simulink model "dropletdet"  (R2012b)
settings: Solver=ode45  SolverMode=SingleTasking  StartTime=0.0  StopTime=43002  RelTol=1e-3
libraries: xbsIndex_r4 x253, simulink x1
(part 1 of 2)
settings Model: Creator=skhay  LastModifiedBy=casrm

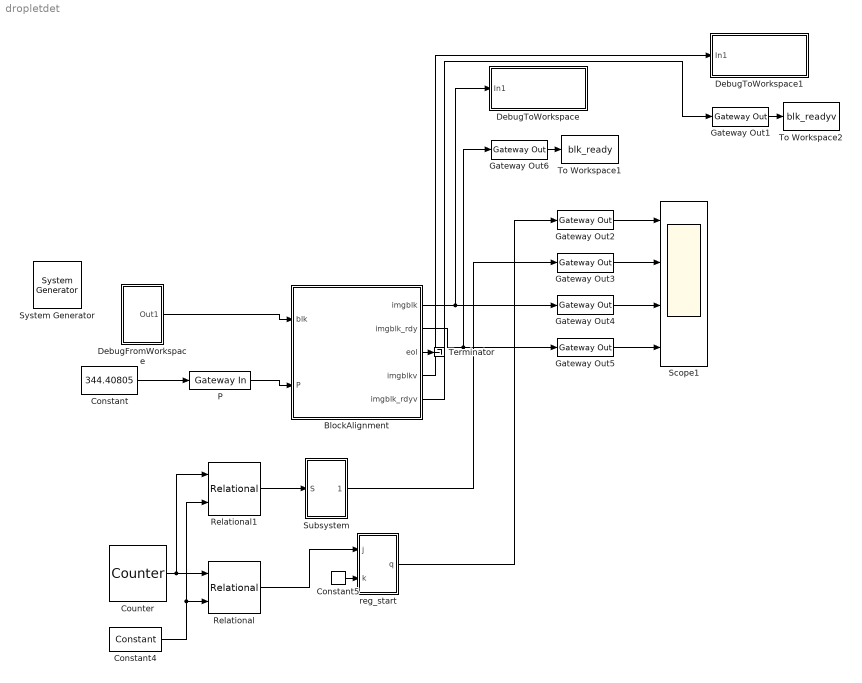
== system dropletdet ==
  " System Generator" : xbsIndex_r4/ System Generator  Tag=genX  xilinxfamily=virtex6  part=xc6vsx475t  speed=-1  package=ff1759  synthesis_tool=XST  clock_wrapper=Clock Enables  directory=./celldet_ppp_sysgen  proj_type=Project Navigator  Synth_file=XST Defaults  Impl_file=ISE Defaults  testbench=off  simulink_period=1  sysclk_period=5  dcm_input_clock_period=100  incr_netlist=off  trim_vbits=Everywhere in SubSystem  dbl_ovrd=According to Block Masks  core_generation=According to Block Masks  run_coregen=off  deprecated_control=off  eval_field=0  block_type=sysgen
      settings: block_version=11.4
  BlockAlignment : Subsystem
  Constant : Constant  Value=344.40805
  Constant4 : xbsIndex_r4/Constant  const=100  gui_display_data_type=Fixed-point  arith_type=Unsigned  n_bits=8  bin_pt=0  preci_type=Single  exp_width=8  frac_width=24  explicit_period=off  period=1  equ=P=C  opselect=C  inp2=PCIN>>17  opr=+  inp1=P  carry=CIN  dbl_ovrd=off  block_type=constant
  Constant5 : xbsIndex_r4/Constant  const=0  gui_display_data_type=Boolean  arith_type=Boolean  n_bits=16  bin_pt=14  preci_type=Single  exp_width=8  frac_width=24  explicit_period=off  period=1  equ=P=C  opselect=C  inp2=PCIN>>17  opr=+  inp1=P  carry=CIN  dbl_ovrd=off  block_type=constant
  Counter : xbsIndex_r4/Counter  cnt_type=Free Running  cnt_to=255  operation=Up  start_count=0  cnt_by_val=1  arith_type=Unsigned  n_bits=8  bin_pt=0  load_pin=off  rst=off  en=off  explicit_period=on  period=1  dbl_ovrd=off  use_behavioral_HDL=off  implementation=Fabric  block_type=counter
  DebugFromWorkspace : Subsystem
  DebugToWorkspace : Subsystem
  DebugToWorkspace1 : Subsystem
  Gateway Out1 : xbsIndex_r4/Gateway Out  inherit_from_input=on  hdl_port=off  timing_constraint=None  locs_specified=off  LOCs={}  UseAsDAC=off  DACChannel='1'  block_type=gatewayout
  Gateway Out{2..5} (4 alike) : xbsIndex_r4/Gateway Out  inherit_from_input=off  hdl_port=off  timing_constraint=None  locs_specified=off  LOCs={}  UseAsDAC=off  DACChannel='1'  block_type=gatewayout
  Gateway Out6 : xbsIndex_r4/Gateway Out  inherit_from_input=on  hdl_port=off  timing_constraint=None  locs_specified=off  LOCs={}  UseAsDAC=off  DACChannel='1'  block_type=gatewayout
  P : xbsIndex_r4/Gateway In  gui_display_data_type=Fixed-point  arith_type=Unsigned  n_bits=32  bin_pt=20  preci_type=Single  exp_width=8  frac_width=24  quantization="Round  (unbiased: +/- Inf)"  overflow=Saturate  period=1  dbl_ovrd=off  timing_constraint=None  locs_specified=off  LOCs={}  UseAsADC=off  ADCChannel='1'  inherit_from_input=off  hdl_port=on  block_type=gatewayin
  Relational : xbsIndex_r4/Relational  mode=a>b  en=off  latency=0  dbl_ovrd=off  block_type=relational
  Relational1 : xbsIndex_r4/Relational  mode=a=b  en=off  latency=0  dbl_ovrd=off  block_type=relational
  Scope1 : Scope  NumInputPorts=4
      settings: YMin=-5~-5~-5~-5  YMax=5~5~5~5  SaveName=ScopeData7
  Subsystem : Subsystem
  Terminator : Terminator
  To Workspace1 : ToWorkspace  VariableName=blk_ready  SampleTime=-1
  To Workspace2 : ToWorkspace  VariableName=blk_readyv  SampleTime=-1
  reg_start : Subsystem
  wires:
  P/1 -> BlockAlignment/2(P)
  Constant/1 -> P/1
  DebugFromWorkspace/1(Out1) -> BlockAlignment/1(blk)
  BlockAlignment/1(imgblk) -> DebugToWorkspace/1(In1), Gateway Out4/1
  BlockAlignment/2(imgblk_rdy) -> Gateway Out6/1, Gateway Out5/1
  BlockAlignment/3(eol) -> Terminator/1
  Counter/1 -> Relational1/1, Relational/1
  Constant4/1 -> Relational1/2, Relational/2
  reg_start/1(q) -> Gateway Out2/1
  Gateway Out5/1 -> Scope1/4
  Gateway Out4/1 -> Scope1/3
  Gateway Out3/1 -> Scope1/2
  Gateway Out2/1 -> Scope1/1
  Relational/1 -> reg_start/1(j)
  Constant5/1 -> reg_start/2(k)
  Subsystem/1(start) -> Gateway Out3/1
  Relational1/1 -> Subsystem/1(S)
  Gateway Out6/1 -> To Workspace1/1
  BlockAlignment/4(imgblkv) -> DebugToWorkspace1/1(In1)
  BlockAlignment/5(imgblk_rdyv) -> Gateway Out1/1
  Gateway Out1/1 -> To Workspace2/1

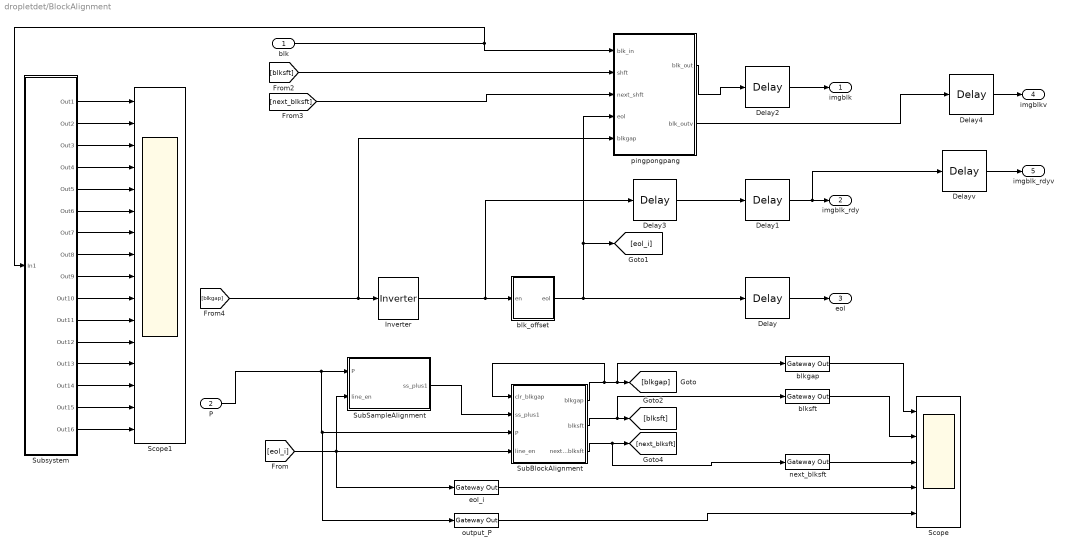
== system dropletdet/BlockAlignment ==
  blk : Inport
  P : Inport  Port=2
  Delay{,1..4} (5 alike) : xbsIndex_r4/Delay  rst=off  infoeditControl=Selection of Reset will increase slice count due to use of real FFs and instead of SRLs  en=off  latency=1  dbl_ovrd=off  reg_retiming=off  block_type=delay
  Delayv : xbsIndex_r4/Delay  rst=off  infoeditControl=Selection of Reset will increase slice count due to use of real FFs and instead of SRLs  en=off  latency=10  dbl_ovrd=off  reg_retiming=off  block_type=delay
  Inverter : xbsIndex_r4/Inverter  en=off  latency=0  dbl_ovrd=off  block_type=inv
  Scope : Scope  NumInputPorts=5
      settings: ShowLegends=on  TimeRange=2102  YMin=-5~-5~-5~-5~-5  YMax=5~5~20~5~5  SaveName=ScopeData4
  Scope1 : Scope  NumInputPorts=16
      settings: TimeRange=2102  YMin=-5~-5~-5~-5~-5~-5~-5~-5~-5~-5~-5~-5~-5~-5~-5~-5  YMax=5~5~20~5~5~5~5~5~5~5~5~5~5~5~5~5  SaveName=ScopeData6
  SubBlockAlignment : Subsystem
  SubSampleAlignment : Subsystem
  Subsystem : Subsystem
  blk_offset : Subsystem
  blkgap : xbsIndex_r4/Gateway Out  inherit_from_input=off  hdl_port=off  timing_constraint=None  locs_specified=off  LOCs={}  UseAsDAC=off  DACChannel='1'  block_type=gatewayout
  blksft : xbsIndex_r4/Gateway Out  inherit_from_input=off  hdl_port=off  timing_constraint=None  locs_specified=off  LOCs={}  UseAsDAC=off  DACChannel='1'  block_type=gatewayout
  eol_i : xbsIndex_r4/Gateway Out  inherit_from_input=off  hdl_port=off  timing_constraint=None  locs_specified=off  LOCs={}  UseAsDAC=off  DACChannel='1'  block_type=gatewayout
  next_blksft : xbsIndex_r4/Gateway Out  inherit_from_input=off  hdl_port=off  timing_constraint=None  locs_specified=off  LOCs={}  UseAsDAC=off  DACChannel='1'  block_type=gatewayout
  output_P : xbsIndex_r4/Gateway Out  inherit_from_input=off  hdl_port=off  timing_constraint=None  locs_specified=off  LOCs={}  UseAsDAC=off  DACChannel='1'  block_type=gatewayout
  pingpongpang : Subsystem
  imgblk : Outport
  imgblk_rdy : Outport  Port=2
  eol : Outport  Port=3
  imgblkv : Outport  Port=4
  imgblk_rdyv : Outport  Port=5
  wires:
  [blkgap] -> pingpongpang/5(blkgap), Inverter/1
  Delay/1 -> eol/1
  [blksft] -> pingpongpang/2(shft)
  [next_blksft] -> pingpongpang/3(next_shft)
  P/1 -> output_P/1, SubBlockAlignment/3(P), SubSampleAlignment/1(P)
  SubSampleAlignment/1(ss_plus1) -> SubBlockAlignment/2(ss_plus1)
  SubBlockAlignment/1(blkgap) -> SubBlockAlignment/1(clr_blkgap), blkgap/1, [blkgap]
  SubBlockAlignment/2(blksft) -> blksft/1, [blksft]
  SubBlockAlignment/3(next_blksft) -> next_blksft/1, [next_blksft]
  [eol_i] -> eol_i/1, SubSampleAlignment/2(line_en), SubBlockAlignment/4(line_en)
  blk/1 -> Subsystem/1(In1), pingpongpang/1(blk_in)
  Delay2/1 -> imgblk/1
  blk_offset/1(eol) -> pingpongpang/4(eol), [eol_i], Delay/1
  Delay1/1 -> Delayv/1, imgblk_rdy/1
  blkgap/1 -> Scope/1
  blksft/1 -> Scope/2
  next_blksft/1 -> Scope/3
  eol_i/1 -> Scope/4
  Inverter/1 -> Delay3/1, blk_offset/1(en)
  Delay3/1 -> Delay1/1
  Subsystem/1(Out1) -> Scope1/1
  Subsystem/2(Out2) -> Scope1/2
  Subsystem/3(Out3) -> Scope1/3
  Subsystem/4(Out4) -> Scope1/4
  Subsystem/5(Out5) -> Scope1/5
  Subsystem/6(Out6) -> Scope1/6
  Subsystem/7(Out7) -> Scope1/7
  Subsystem/8(Out8) -> Scope1/8
  Subsystem/9(Out9) -> Scope1/9
  Subsystem/10(Out10) -> Scope1/10
  Subsystem/11(Out11) -> Scope1/11
  Subsystem/12(Out12) -> Scope1/12
  Subsystem/13(Out13) -> Scope1/13
  Subsystem/14(Out14) -> Scope1/14
  Subsystem/15(Out15) -> Scope1/15
  Subsystem/16(Out16) -> Scope1/16
  output_P/1 -> Scope/5
  Delay4/1 -> imgblkv/1
  pingpongpang/1(blk_out) -> Delay2/1
  Delayv/1 -> imgblk_rdyv/1
  pingpongpang/2(blk_outv) -> Delay4/1

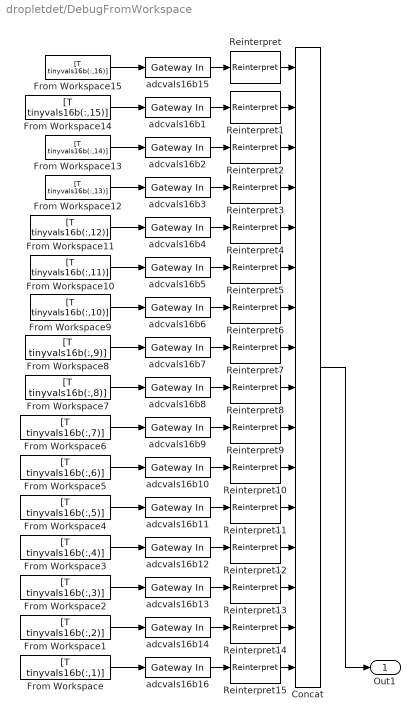
== system dropletdet/DebugFromWorkspace ==
  Concat : xbsIndex_r4/Concat  num_inputs=16  dbl_ovrd=off  block_type=concat
  From Workspace : FromWorkspace  VariableName=[T tinyvals16b(:,1)]  SampleTime=1
  From Workspace1 : FromWorkspace  VariableName=[T tinyvals16b(:,2)]  SampleTime=1
  From Workspace10 : FromWorkspace  VariableName=[T tinyvals16b(:,11)]  SampleTime=1
  From Workspace11 : FromWorkspace  VariableName=[T tinyvals16b(:,12)]  SampleTime=1
  From Workspace12 : FromWorkspace  VariableName=[T tinyvals16b(:,13)]  SampleTime=1
  From Workspace13 : FromWorkspace  VariableName=[T tinyvals16b(:,14)]  SampleTime=1
  From Workspace14 : FromWorkspace  VariableName=[T tinyvals16b(:,15)]  SampleTime=1
  From Workspace15 : FromWorkspace  VariableName=[T tinyvals16b(:,16)]  SampleTime=1
  From Workspace2 : FromWorkspace  VariableName=[T tinyvals16b(:,3)]  SampleTime=1
  From Workspace3 : FromWorkspace  VariableName=[T tinyvals16b(:,4)]  SampleTime=1
  From Workspace4 : FromWorkspace  VariableName=[T tinyvals16b(:,5)]  SampleTime=1
  From Workspace5 : FromWorkspace  VariableName=[T tinyvals16b(:,6)]  SampleTime=1
  From Workspace6 : FromWorkspace  VariableName=[T tinyvals16b(:,7)]  SampleTime=1
  From Workspace7 : FromWorkspace  VariableName=[T tinyvals16b(:,8)]  SampleTime=1
  From Workspace8 : FromWorkspace  VariableName=[T tinyvals16b(:,9)]  SampleTime=1
  From Workspace9 : FromWorkspace  VariableName=[T tinyvals16b(:,10)]  SampleTime=1
  Reinterpret{,1..15} (16 alike) : xbsIndex_r4/Reinterpret  force_arith_type=on  arith_type=Unsigned  force_bin_pt=on  bin_pt=0  block_type=reinterpret
  adcvals16b{1..16} (16 alike) : xbsIndex_r4/Gateway In  gui_display_data_type=Fixed-point  arith_type="Signed  (2's comp)"  n_bits=8  bin_pt=0  preci_type=Single  exp_width=8  frac_width=24  quantization="Round  (unbiased: +/- Inf)"  overflow=Saturate  period=1  dbl_ovrd=off  timing_constraint=None  locs_specified=off  LOCs={}  UseAsADC=off  ADCChannel='1'  inherit_from_input=off  hdl_port=on  block_type=gatewayin
  Out1 : Outport
  wires:
  Concat/1 -> Out1/1
  From Workspace15/1 -> adcvals16b15/1
  From Workspace14/1 -> adcvals16b1/1
  From Workspace13/1 -> adcvals16b2/1
  From Workspace12/1 -> adcvals16b3/1
  From Workspace11/1 -> adcvals16b4/1
  From Workspace10/1 -> adcvals16b5/1
  From Workspace9/1 -> adcvals16b6/1
  From Workspace8/1 -> adcvals16b7/1
  From Workspace7/1 -> adcvals16b8/1
  From Workspace6/1 -> adcvals16b9/1
  From Workspace5/1 -> adcvals16b10/1
  From Workspace4/1 -> adcvals16b11/1
  From Workspace3/1 -> adcvals16b12/1
  From Workspace2/1 -> adcvals16b13/1
  From Workspace1/1 -> adcvals16b14/1
  From Workspace/1 -> adcvals16b16/1
  adcvals16b15/1 -> Reinterpret/1
  Reinterpret/1 -> Concat/1
  adcvals16b1/1 -> Reinterpret1/1
  Reinterpret1/1 -> Concat/2
  adcvals16b2/1 -> Reinterpret2/1
  Reinterpret2/1 -> Concat/3
  adcvals16b3/1 -> Reinterpret3/1
  Reinterpret3/1 -> Concat/4
  adcvals16b4/1 -> Reinterpret4/1
  Reinterpret4/1 -> Concat/5
  adcvals16b5/1 -> Reinterpret5/1
  Reinterpret5/1 -> Concat/6
  adcvals16b6/1 -> Reinterpret6/1
  Reinterpret6/1 -> Concat/7
  adcvals16b7/1 -> Reinterpret7/1
  Reinterpret7/1 -> Concat/8
  adcvals16b8/1 -> Reinterpret8/1
  Reinterpret8/1 -> Concat/9
  adcvals16b9/1 -> Reinterpret9/1
  Reinterpret9/1 -> Concat/10
  adcvals16b10/1 -> Reinterpret10/1
  Reinterpret10/1 -> Concat/11
  adcvals16b11/1 -> Reinterpret11/1
  Reinterpret11/1 -> Concat/12
  adcvals16b12/1 -> Reinterpret12/1
  Reinterpret12/1 -> Concat/13
  adcvals16b13/1 -> Reinterpret13/1
  Reinterpret13/1 -> Concat/14
  adcvals16b14/1 -> Reinterpret14/1
  Reinterpret14/1 -> Concat/15
  adcvals16b16/1 -> Reinterpret15/1
  Reinterpret15/1 -> Concat/16

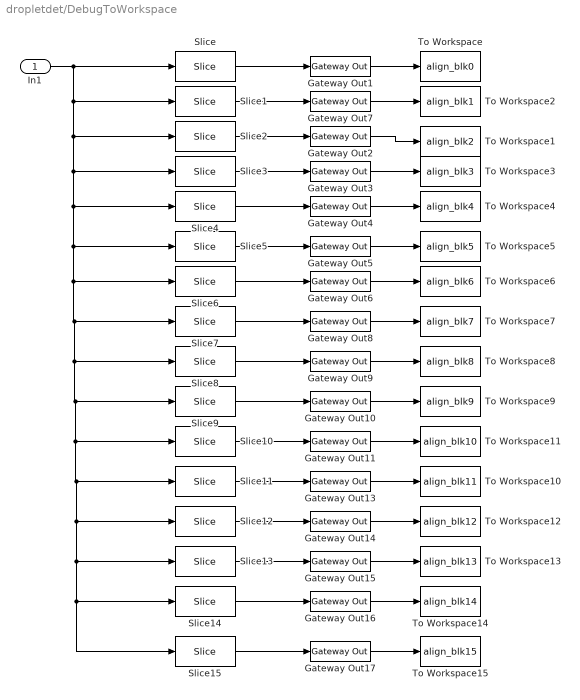
== system dropletdet/DebugToWorkspace ==
  In1 : Inport
  Gateway Out{1..11,13..17} (16 alike) : xbsIndex_r4/Gateway Out  inherit_from_input=on  hdl_port=off  timing_constraint=None  locs_specified=off  LOCs={}  UseAsDAC=off  DACChannel='1'  block_type=gatewayout
  Slice : xbsIndex_r4/Slice  nbits=8  boolean_output=off  mode=Lower Bit Location + Width  bit1=120  base1=MSB of Input  bit0=0  base0=LSB of Input  dbl_ovrd=off  block_type=slice
  Slice1 : xbsIndex_r4/Slice  nbits=8  boolean_output=off  mode=Lower Bit Location + Width  bit1=120  base1=MSB of Input  bit0=8  base0=LSB of Input  dbl_ovrd=off  block_type=slice
  Slice10 : xbsIndex_r4/Slice  nbits=8  boolean_output=off  mode=Lower Bit Location + Width  bit1=120  base1=MSB of Input  bit0=80  base0=LSB of Input  dbl_ovrd=off  block_type=slice
  Slice11 : xbsIndex_r4/Slice  nbits=8  boolean_output=off  mode=Lower Bit Location + Width  bit1=120  base1=MSB of Input  bit0=88  base0=LSB of Input  dbl_ovrd=off  block_type=slice
  Slice12 : xbsIndex_r4/Slice  nbits=8  boolean_output=off  mode=Lower Bit Location + Width  bit1=120  base1=MSB of Input  bit0=96  base0=LSB of Input  dbl_ovrd=off  block_type=slice
  Slice13 : xbsIndex_r4/Slice  nbits=8  boolean_output=off  mode=Lower Bit Location + Width  bit1=120  base1=MSB of Input  bit0=104  base0=LSB of Input  dbl_ovrd=off  block_type=slice
  Slice14 : xbsIndex_r4/Slice  nbits=8  boolean_output=off  mode=Lower Bit Location + Width  bit1=120  base1=MSB of Input  bit0=112  base0=LSB of Input  dbl_ovrd=off  block_type=slice
  Slice15 : xbsIndex_r4/Slice  nbits=8  boolean_output=off  mode=Lower Bit Location + Width  bit1=120  base1=MSB of Input  bit0=120  base0=LSB of Input  dbl_ovrd=off  block_type=slice
  Slice2 : xbsIndex_r4/Slice  nbits=8  boolean_output=off  mode=Lower Bit Location + Width  bit1=120  base1=MSB of Input  bit0=16  base0=LSB of Input  dbl_ovrd=off  block_type=slice
  Slice3 : xbsIndex_r4/Slice  nbits=8  boolean_output=off  mode=Lower Bit Location + Width  bit1=120  base1=MSB of Input  bit0=24  base0=LSB of Input  dbl_ovrd=off  block_type=slice
  Slice4 : xbsIndex_r4/Slice  nbits=8  boolean_output=off  mode=Lower Bit Location + Width  bit1=120  base1=MSB of Input  bit0=32  base0=LSB of Input  dbl_ovrd=off  block_type=slice
  Slice5 : xbsIndex_r4/Slice  nbits=8  boolean_output=off  mode=Lower Bit Location + Width  bit1=120  base1=MSB of Input  bit0=40  base0=LSB of Input  dbl_ovrd=off  block_type=slice
  Slice6 : xbsIndex_r4/Slice  nbits=8  boolean_output=off  mode=Lower Bit Location + Width  bit1=120  base1=MSB of Input  bit0=48  base0=LSB of Input  dbl_ovrd=off  block_type=slice
  Slice7 : xbsIndex_r4/Slice  nbits=8  boolean_output=off  mode=Lower Bit Location + Width  bit1=120  base1=MSB of Input  bit0=56  base0=LSB of Input  dbl_ovrd=off  block_type=slice
  Slice8 : xbsIndex_r4/Slice  nbits=8  boolean_output=off  mode=Lower Bit Location + Width  bit1=120  base1=MSB of Input  bit0=64  base0=LSB of Input  dbl_ovrd=off  block_type=slice
  Slice9 : xbsIndex_r4/Slice  nbits=8  boolean_output=off  mode=Lower Bit Location + Width  bit1=120  base1=MSB of Input  bit0=72  base0=LSB of Input  dbl_ovrd=off  block_type=slice
  To Workspace : ToWorkspace  VariableName=align_blk0  SampleTime=-1
  To Workspace1 : ToWorkspace  VariableName=align_blk2  SampleTime=-1
  To Workspace10 : ToWorkspace  VariableName=align_blk11  SampleTime=-1
  To Workspace11 : ToWorkspace  VariableName=align_blk10  SampleTime=-1
  To Workspace12 : ToWorkspace  VariableName=align_blk12  SampleTime=-1
  To Workspace13 : ToWorkspace  VariableName=align_blk13  SampleTime=-1
  To Workspace14 : ToWorkspace  VariableName=align_blk14  SampleTime=-1
  To Workspace15 : ToWorkspace  VariableName=align_blk15  SampleTime=-1
  To Workspace2 : ToWorkspace  VariableName=align_blk1  SampleTime=-1
  To Workspace3 : ToWorkspace  VariableName=align_blk3  SampleTime=-1
  To Workspace4 : ToWorkspace  VariableName=align_blk4  SampleTime=-1
  To Workspace5 : ToWorkspace  VariableName=align_blk5  SampleTime=-1
  To Workspace6 : ToWorkspace  VariableName=align_blk6  SampleTime=-1
  To Workspace7 : ToWorkspace  VariableName=align_blk7  SampleTime=-1
  To Workspace8 : ToWorkspace  VariableName=align_blk8  SampleTime=-1
  To Workspace9 : ToWorkspace  VariableName=align_blk9  SampleTime=-1
  wires:
  Gateway Out1/1 -> To Workspace/1
  Slice/1 -> Gateway Out1/1
  Gateway Out7/1 -> To Workspace2/1
  Slice1/1 -> Gateway Out7/1
  Gateway Out2/1 -> To Workspace1/1
  Slice2/1 -> Gateway Out2/1
  Gateway Out3/1 -> To Workspace3/1
  Slice3/1 -> Gateway Out3/1
  Gateway Out4/1 -> To Workspace4/1
  Slice4/1 -> Gateway Out4/1
  Gateway Out5/1 -> To Workspace5/1
  Slice5/1 -> Gateway Out5/1
  Gateway Out6/1 -> To Workspace6/1
  Slice6/1 -> Gateway Out6/1
  Gateway Out8/1 -> To Workspace7/1
  Slice7/1 -> Gateway Out8/1
  Gateway Out9/1 -> To Workspace8/1
  Slice8/1 -> Gateway Out9/1
  Slice9/1 -> Gateway Out10/1
  Gateway Out11/1 -> To Workspace11/1
  Slice10/1 -> Gateway Out11/1
  Gateway Out13/1 -> To Workspace10/1
  Slice11/1 -> Gateway Out13/1
  Gateway Out14/1 -> To Workspace12/1
  Slice12/1 -> Gateway Out14/1
  Gateway Out15/1 -> To Workspace13/1
  Slice13/1 -> Gateway Out15/1
  Gateway Out16/1 -> To Workspace14/1
  Slice14/1 -> Gateway Out16/1
  Gateway Out17/1 -> To Workspace15/1
  Slice15/1 -> Gateway Out17/1
  In1/1 -> Slice15/1, Slice14/1, Slice13/1, Slice12/1, Slice11/1, Slice10/1, Slice9/1, Slice8/1, Slice7/1, Slice6/1, Slice5/1, Slice4/1, Slice3/1, Slice2/1, Slice1/1, Slice/1
  Gateway Out10/1 -> To Workspace9/1

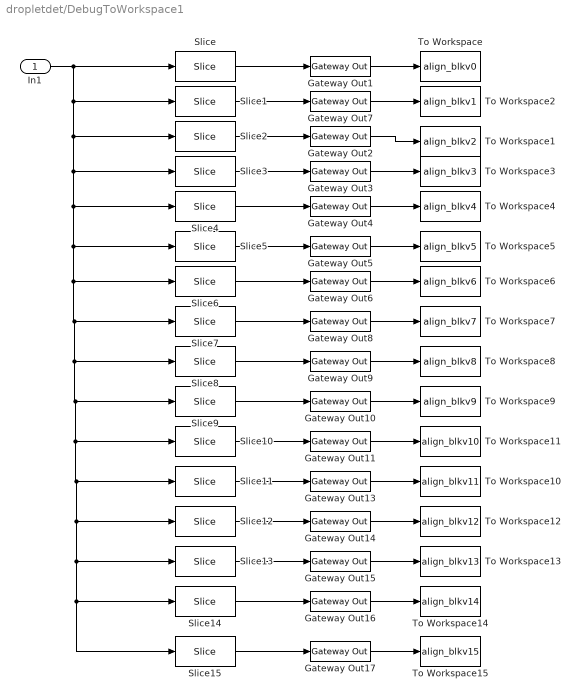
== system dropletdet/DebugToWorkspace1 ==
  In1 : Inport
  Gateway Out{1..11,13..17} (16 alike) : xbsIndex_r4/Gateway Out  inherit_from_input=on  hdl_port=off  timing_constraint=None  locs_specified=off  LOCs={}  UseAsDAC=off  DACChannel='1'  block_type=gatewayout
  Slice : xbsIndex_r4/Slice  nbits=8  boolean_output=off  mode=Lower Bit Location + Width  bit1=120  base1=MSB of Input  bit0=0  base0=LSB of Input  dbl_ovrd=off  block_type=slice
  Slice1 : xbsIndex_r4/Slice  nbits=8  boolean_output=off  mode=Lower Bit Location + Width  bit1=120  base1=MSB of Input  bit0=8  base0=LSB of Input  dbl_ovrd=off  block_type=slice
  Slice10 : xbsIndex_r4/Slice  nbits=8  boolean_output=off  mode=Lower Bit Location + Width  bit1=120  base1=MSB of Input  bit0=80  base0=LSB of Input  dbl_ovrd=off  block_type=slice
  Slice11 : xbsIndex_r4/Slice  nbits=8  boolean_output=off  mode=Lower Bit Location + Width  bit1=120  base1=MSB of Input  bit0=88  base0=LSB of Input  dbl_ovrd=off  block_type=slice
  Slice12 : xbsIndex_r4/Slice  nbits=8  boolean_output=off  mode=Lower Bit Location + Width  bit1=120  base1=MSB of Input  bit0=96  base0=LSB of Input  dbl_ovrd=off  block_type=slice
  Slice13 : xbsIndex_r4/Slice  nbits=8  boolean_output=off  mode=Lower Bit Location + Width  bit1=120  base1=MSB of Input  bit0=104  base0=LSB of Input  dbl_ovrd=off  block_type=slice
  Slice14 : xbsIndex_r4/Slice  nbits=8  boolean_output=off  mode=Lower Bit Location + Width  bit1=120  base1=MSB of Input  bit0=112  base0=LSB of Input  dbl_ovrd=off  block_type=slice
  Slice15 : xbsIndex_r4/Slice  nbits=8  boolean_output=off  mode=Lower Bit Location + Width  bit1=120  base1=MSB of Input  bit0=120  base0=LSB of Input  dbl_ovrd=off  block_type=slice
  Slice2 : xbsIndex_r4/Slice  nbits=8  boolean_output=off  mode=Lower Bit Location + Width  bit1=120  base1=MSB of Input  bit0=16  base0=LSB of Input  dbl_ovrd=off  block_type=slice
  Slice3 : xbsIndex_r4/Slice  nbits=8  boolean_output=off  mode=Lower Bit Location + Width  bit1=120  base1=MSB of Input  bit0=24  base0=LSB of Input  dbl_ovrd=off  block_type=slice
  Slice4 : xbsIndex_r4/Slice  nbits=8  boolean_output=off  mode=Lower Bit Location + Width  bit1=120  base1=MSB of Input  bit0=32  base0=LSB of Input  dbl_ovrd=off  block_type=slice
  Slice5 : xbsIndex_r4/Slice  nbits=8  boolean_output=off  mode=Lower Bit Location + Width  bit1=120  base1=MSB of Input  bit0=40  base0=LSB of Input  dbl_ovrd=off  block_type=slice
  Slice6 : xbsIndex_r4/Slice  nbits=8  boolean_output=off  mode=Lower Bit Location + Width  bit1=120  base1=MSB of Input  bit0=48  base0=LSB of Input  dbl_ovrd=off  block_type=slice
  Slice7 : xbsIndex_r4/Slice  nbits=8  boolean_output=off  mode=Lower Bit Location + Width  bit1=120  base1=MSB of Input  bit0=56  base0=LSB of Input  dbl_ovrd=off  block_type=slice
  Slice8 : xbsIndex_r4/Slice  nbits=8  boolean_output=off  mode=Lower Bit Location + Width  bit1=120  base1=MSB of Input  bit0=64  base0=LSB of Input  dbl_ovrd=off  block_type=slice
  Slice9 : xbsIndex_r4/Slice  nbits=8  boolean_output=off  mode=Lower Bit Location + Width  bit1=120  base1=MSB of Input  bit0=72  base0=LSB of Input  dbl_ovrd=off  block_type=slice
  To Workspace : ToWorkspace  VariableName=align_blkv0  SampleTime=-1
  To Workspace1 : ToWorkspace  VariableName=align_blkv2  SampleTime=-1
  To Workspace10 : ToWorkspace  VariableName=align_blkv11  SampleTime=-1
  To Workspace11 : ToWorkspace  VariableName=align_blkv10  SampleTime=-1
  To Workspace12 : ToWorkspace  VariableName=align_blkv12  SampleTime=-1
  To Workspace13 : ToWorkspace  VariableName=align_blkv13  SampleTime=-1
  To Workspace14 : ToWorkspace  VariableName=align_blkv14  SampleTime=-1
  To Workspace15 : ToWorkspace  VariableName=align_blkv15  SampleTime=-1
  To Workspace2 : ToWorkspace  VariableName=align_blkv1  SampleTime=-1
  To Workspace3 : ToWorkspace  VariableName=align_blkv3  SampleTime=-1
  To Workspace4 : ToWorkspace  VariableName=align_blkv4  SampleTime=-1
  To Workspace5 : ToWorkspace  VariableName=align_blkv5  SampleTime=-1
  To Workspace6 : ToWorkspace  VariableName=align_blkv6  SampleTime=-1
  To Workspace7 : ToWorkspace  VariableName=align_blkv7  SampleTime=-1
  To Workspace8 : ToWorkspace  VariableName=align_blkv8  SampleTime=-1
  To Workspace9 : ToWorkspace  VariableName=align_blkv9  SampleTime=-1
  wires:
  Gateway Out10/1 -> To Workspace9/1
  In1/1 -> Slice/1, Slice1/1, Slice2/1, Slice3/1, Slice4/1, Slice5/1, Slice6/1, Slice7/1, Slice8/1, Slice9/1, Slice10/1, Slice11/1, Slice12/1, Slice13/1, Slice14/1, Slice15/1
  Slice15/1 -> Gateway Out17/1
  Gateway Out17/1 -> To Workspace15/1
  Slice14/1 -> Gateway Out16/1
  Gateway Out16/1 -> To Workspace14/1
  Slice13/1 -> Gateway Out15/1
  Gateway Out15/1 -> To Workspace13/1
  Slice12/1 -> Gateway Out14/1
  Gateway Out14/1 -> To Workspace12/1
  Slice11/1 -> Gateway Out13/1
  Gateway Out13/1 -> To Workspace10/1
  Slice10/1 -> Gateway Out11/1
  Gateway Out11/1 -> To Workspace11/1
  Slice9/1 -> Gateway Out10/1
  Slice8/1 -> Gateway Out9/1
  Gateway Out9/1 -> To Workspace8/1
  Slice7/1 -> Gateway Out8/1
  Gateway Out8/1 -> To Workspace7/1
  Slice6/1 -> Gateway Out6/1
  Gateway Out6/1 -> To Workspace6/1
  Slice5/1 -> Gateway Out5/1
  Gateway Out5/1 -> To Workspace5/1
  Slice4/1 -> Gateway Out4/1
  Gateway Out4/1 -> To Workspace4/1
  Slice3/1 -> Gateway Out3/1
  Gateway Out3/1 -> To Workspace3/1
  Slice2/1 -> Gateway Out2/1
  Gateway Out2/1 -> To Workspace1/1
  Slice1/1 -> Gateway Out7/1
  Gateway Out7/1 -> To Workspace2/1
  Slice/1 -> Gateway Out1/1
  Gateway Out1/1 -> To Workspace/1

== system dropletdet/Subsystem ==
  S : Inport
  Expression : xbsIndex_r4/Expression  expression=s | s0 | s1  align_bp=off  en=off  latency=0  precision=Full  arith_type=Unsigned  n_bits=16  bin_pt=0  dbl_ovrd=off  block_type=expr
  Expression1 : xbsIndex_r4/Expression  expression=s0 & ~s1  align_bp=off  en=off  latency=0  precision=Full  arith_type=Unsigned  n_bits=16  bin_pt=0  dbl_ovrd=off  block_type=expr
  Expression2 : xbsIndex_r4/Expression  expression=s0 | s1  align_bp=off  en=off  latency=0  precision=Full  arith_type=Unsigned  n_bits=16  bin_pt=0  dbl_ovrd=off  block_type=expr
  Register1 : xbsIndex_r4/Register  init=0  rst=off  en=off  dbl_ovrd=off  block_type=register
  Register2 : xbsIndex_r4/Register  init=0  rst=off  en=off  dbl_ovrd=off  block_type=register
  start : Outport
  wires:
  Expression1/1 -> start/1
  S/1 -> Expression/1
  Register1/1 -> Expression/2, Expression2/1, Expression1/1
  Expression2/1 -> Register2/1
  Register2/1 -> Expression2/2, Expression/3, Expression1/2
  Expression/1 -> Register1/1

== system dropletdet/reg_start ==
  j : Inport
  k : Inport  Port=2
  Expression : xbsIndex_r4/Expression  expression=(~q & j) | (q & ~k)  align_bp=off  en=off  latency=0  precision=Full  arith_type=Unsigned  n_bits=16  bin_pt=0  dbl_ovrd=off  block_type=expr
  Register1 : xbsIndex_r4/Register  init=0  rst=off  en=off  dbl_ovrd=off  block_type=register
  q : Outport
  wires:
  Register1/1 -> Expression/3, q/1
  Expression/1 -> Register1/1
  k/1 -> Expression/2
  j/1 -> Expression/1

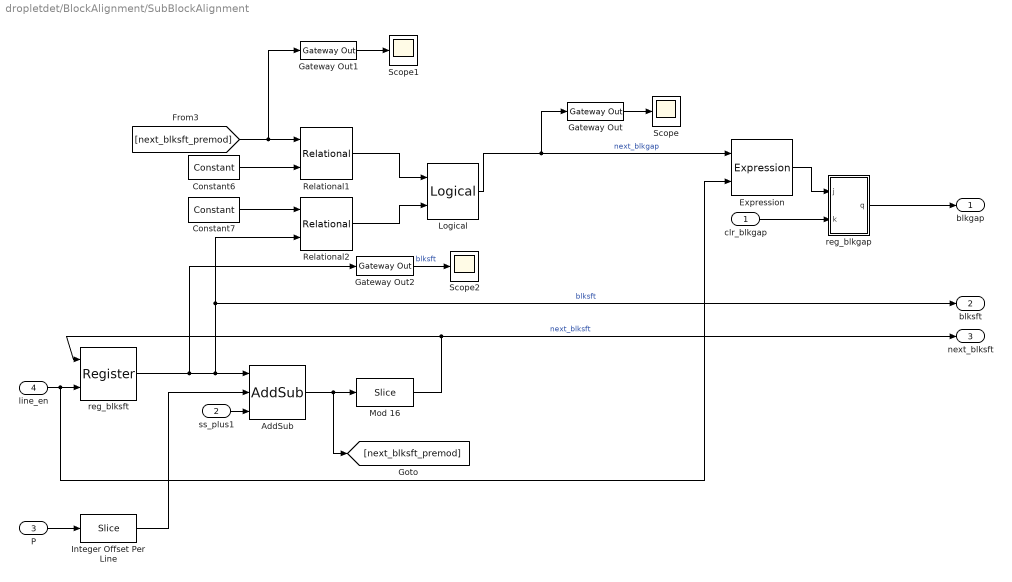
== system dropletdet/BlockAlignment/SubBlockAlignment ==
  clr_blkgap : Inport
  ss_plus1 : Inport  Port=2
  P : Inport  Port=3
  line_en : Inport  Port=4
  AddSub : xbsIndex_r4/AddSub  mode=Addition  use_carryin=on  use_carryout=off  en=off  latency=0  precision=Full  arith_type=Unsigned  n_bits=16  bin_pt=14  quantization=Truncate  overflow=Wrap  dbl_ovrd=off  use_behavioral_HDL=off  hw_selection=Fabric  pipelined=off  block_type=addsub
  Constant6 : xbsIndex_r4/Constant  const=16  gui_display_data_type=Fixed-point  arith_type=Unsigned  n_bits=5  bin_pt=0  preci_type=Single  exp_width=8  frac_width=24  explicit_period=off  period=1  equ=P=C  opselect=C  inp2=PCIN>>17  opr=+  inp1=P  carry=CIN  dbl_ovrd=off  block_type=constant
  Constant7 : xbsIndex_r4/Constant  const=0  gui_display_data_type=Fixed-point  arith_type=Unsigned  n_bits=5  bin_pt=0  preci_type=Single  exp_width=8  frac_width=24  explicit_period=off  period=1  equ=P=C  opselect=C  inp2=PCIN>>17  opr=+  inp1=P  carry=CIN  dbl_ovrd=off  block_type=constant
  Expression : xbsIndex_r4/Expression  expression=a & b  align_bp=on  en=off  latency=0  precision=Full  arith_type=Unsigned  n_bits=16  bin_pt=0  dbl_ovrd=off  block_type=expr
  Gateway Out : xbsIndex_r4/Gateway Out  inherit_from_input=off  hdl_port=on  timing_constraint=None  locs_specified=off  LOCs={}  UseAsDAC=off  DACChannel='1'  block_type=gatewayout
  Gateway Out1 : xbsIndex_r4/Gateway Out  inherit_from_input=off  hdl_port=on  timing_constraint=None  locs_specified=off  LOCs={}  UseAsDAC=off  DACChannel='1'  block_type=gatewayout
  Gateway Out2 : xbsIndex_r4/Gateway Out  inherit_from_input=off  hdl_port=on  timing_constraint=None  locs_specified=off  LOCs={}  UseAsDAC=off  DACChannel='1'  block_type=gatewayout
  Integer Offset Per Line : xbsIndex_r4/Slice  nbits=4  boolean_output=off  mode=Lower Bit Location + Width  bit1=0  base1=MSB of Input  bit0=20  base0=LSB of Input  dbl_ovrd=off  block_type=slice
  Logical : xbsIndex_r4/Logical  logical_function=OR  inputs=2  en=off  latency=0  precision=Full  arith_type=Unsigned  n_bits=16  bin_pt=0  align_bp=on  dbl_ovrd=off  block_type=logical
  Mod 16 : xbsIndex_r4/Slice  nbits=4  boolean_output=off  mode=Lower Bit Location + Width  bit1=1  base1=MSB of Input  bit0=0  base0=LSB of Input  dbl_ovrd=off  block_type=slice
  Relational1 : xbsIndex_r4/Relational  mode=a>b  en=off  latency=0  dbl_ovrd=off  block_type=relational
  Relational2 : xbsIndex_r4/Relational  mode=a=b  en=off  latency=0  dbl_ovrd=off  block_type=relational
  Scope : Scope
  Scope1 : Scope
      settings: SaveName=ScopeData2
  Scope2 : Scope
      settings: SaveName=ScopeData3
  reg_blkgap : Subsystem
  reg_blksft : xbsIndex_r4/Register  init=0  rst=off  en=on  dbl_ovrd=off  block_type=register
  blkgap : Outport
  blksft : Outport  Port=2
  next_blksft : Outport  Port=3
  wires:
  Mod 16/1 -> next_blksft/1, reg_blksft/1  "next_blksft"
  Integer Offset Per Line/1 -> AddSub/2
  AddSub/1 -> [next_blksft_premod], Mod 16/1
  reg_blksft/1 -> Gateway Out2/1, blksft/1, Relational2/2, AddSub/1  "blksft"
  line_en/1 -> Expression/2, reg_blksft/2
  Constant7/1 -> Relational2/1
  clr_blkgap/1 -> reg_blkgap/2(k)
  Logical/1 -> Gateway Out/1, Expression/1  "next_blkgap"
  [next_blksft_premod] -> Gateway Out1/1, Relational1/1
  ss_plus1/1 -> AddSub/3
  reg_blkgap/1(q) -> blkgap/1
  Relational2/1 -> Logical/2
  Constant6/1 -> Relational1/2
  Relational1/1 -> Logical/1
  Gateway Out/1 -> Scope/1
  Gateway Out1/1 -> Scope1/1
  Gateway Out2/1 -> Scope2/1  "blksft"
  Expression/1 -> reg_blkgap/1(j)
  P/1 -> Integer Offset Per Line/1

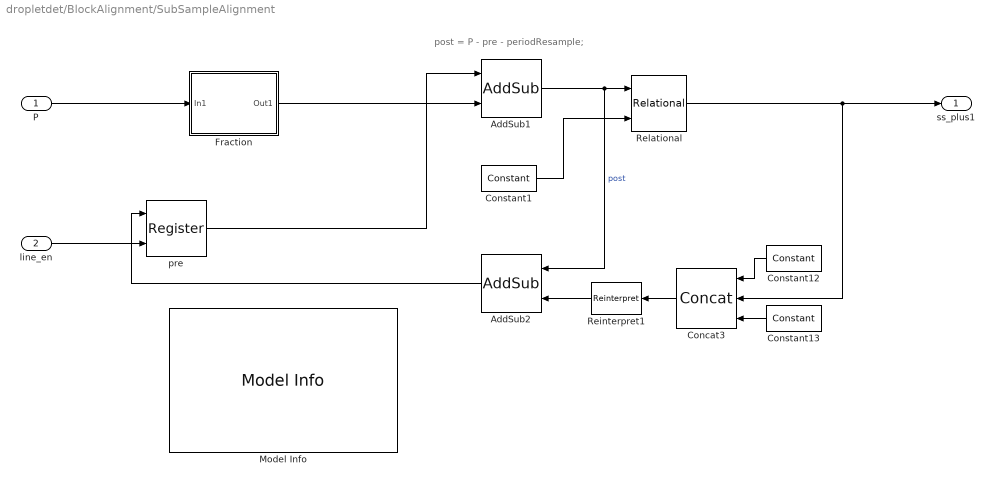
== system dropletdet/BlockAlignment/SubSampleAlignment ==
  note: post = P - pre - periodResample;
  P : Inport
  line_en : Inport  Port=2
  AddSub1 : xbsIndex_r4/AddSub  mode=Subtraction  use_carryin=off  use_carryout=off  en=off  latency=0  precision=User Defined  arith_type="Signed  (2's comp)"  n_bits=22  bin_pt=20  quantization=Truncate  overflow=Wrap  dbl_ovrd=off  use_behavioral_HDL=off  hw_selection=Fabric  pipelined=off  block_type=addsub
  AddSub2 : xbsIndex_r4/AddSub  mode=Addition  use_carryin=off  use_carryout=off  en=off  latency=0  precision=User Defined  arith_type="Signed  (2's comp)"  n_bits=22  bin_pt=20  quantization=Truncate  overflow=Wrap  dbl_ovrd=off  use_behavioral_HDL=off  hw_selection=Fabric  pipelined=off  block_type=addsub
  Concat3 : xbsIndex_r4/Concat  num_inputs=3  dbl_ovrd=off  block_type=concat
  Constant1 : xbsIndex_r4/Constant  const=0  gui_display_data_type=Fixed-point  arith_type=Signed (2's comp)  n_bits=22  bin_pt=20  preci_type=Single  exp_width=8  frac_width=24  explicit_period=off  period=1  equ=P=C  opselect=C  inp2=PCIN>>17  opr=+  inp1=P  carry=CIN  dbl_ovrd=off  block_type=constant
  Constant12 : xbsIndex_r4/Constant  const=0  gui_display_data_type=Fixed-point  arith_type=Unsigned  n_bits=1  bin_pt=0  preci_type=Single  exp_width=8  frac_width=24  explicit_period=off  period=1  equ=P=C  opselect=C  inp2=PCIN>>17  opr=+  inp1=P  carry=CIN  dbl_ovrd=off  block_type=constant
  Constant13 : xbsIndex_r4/Constant  const=0  gui_display_data_type=Fixed-point  arith_type=Unsigned  n_bits=20  bin_pt=0  preci_type=Single  exp_width=8  frac_width=24  explicit_period=off  period=1  equ=P=C  opselect=C  inp2=PCIN>>17  opr=+  inp1=P  carry=CIN  dbl_ovrd=off  block_type=constant
  Fraction : Subsystem
  Model Info : simulink/Model-Wide Utilities/Model Info  InitialBlockCM=None  BlockCM=None  Frame=on  DisplayStringWithTags=|  HorizontalTextAlignment=Left  LeftAlignmentValue=0.02  SourceBlockDiagram=dropletdet  TagMaxNumber=20
      | post = pre - (P - periodResample);
      |     if (post < 0)
      |         % skip 1 more
      |         next_blksft = next_blksft + 1;
      |         pre = 1 + post;
      |     else
      |         % no need to skip
      |         pre = post;
      |     end
  Reinterpret1 : xbsIndex_r4/Reinterpret  force_arith_type=on  arith_type="Signed  (2's comp)"  force_bin_pt=on  bin_pt=20  block_type=reinterpret
  Relational : xbsIndex_r4/Relational  mode=a<b  en=off  latency=0  dbl_ovrd=off  block_type=relational
  pre : xbsIndex_r4/Register  init=0  rst=off  en=on  dbl_ovrd=off  block_type=register
  ss_plus1 : Outport
  wires:
  Relational/1 -> ss_plus1/1, Concat3/2
  Constant1/1 -> Relational/2
  Constant12/1 -> Concat3/1
  Reinterpret1/1 -> AddSub2/2
  Constant13/1 -> Concat3/3
  pre/1 -> AddSub1/1
  AddSub1/1 -> AddSub2/1, Relational/1  "post"
  Concat3/1 -> Reinterpret1/1
  AddSub2/1 -> pre/1
  line_en/1 -> pre/2
  P/1 -> Fraction/1(In1)
  Fraction/1(Out1) -> AddSub1/2

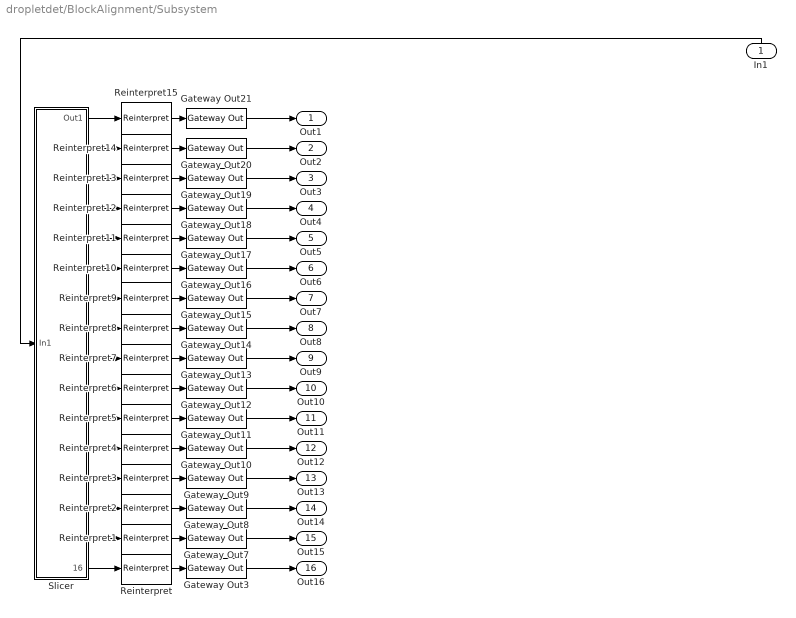
== system dropletdet/BlockAlignment/Subsystem ==
  In1 : Inport
  Gateway Out{3,7..21} (16 alike) : xbsIndex_r4/Gateway Out  inherit_from_input=off  hdl_port=off  timing_constraint=None  locs_specified=off  LOCs={}  UseAsDAC=off  DACChannel='1'  block_type=gatewayout
  Reinterpret{,1..15} (16 alike) : xbsIndex_r4/Reinterpret  force_arith_type=on  arith_type="Signed  (2's comp)"  force_bin_pt=on  bin_pt=0  block_type=reinterpret
  Slicer : Subsystem
  Out1 : Outport
  Out2 : Outport  Port=2
  Out3 : Outport  Port=3
  Out4 : Outport  Port=4
  Out5 : Outport  Port=5
  Out6 : Outport  Port=6
  Out7 : Outport  Port=7
  Out8 : Outport  Port=8
  Out9 : Outport  Port=9
  Out10 : Outport  Port=10
  Out11 : Outport  Port=11
  Out12 : Outport  Port=12
  Out13 : Outport  Port=13
  Out14 : Outport  Port=14
  Out15 : Outport  Port=15
  Out16 : Outport  Port=16
  wires:
  In1/1 -> Slicer/1(In1)
  Slicer/16(Out16) -> Reinterpret/1
  Slicer/15(Out15) -> Reinterpret1/1
  Slicer/14(Out14) -> Reinterpret2/1
  Slicer/13(Out13) -> Reinterpret3/1
  Slicer/12(Out12) -> Reinterpret4/1
  Slicer/11(Out11) -> Reinterpret5/1
  Slicer/10(Out10) -> Reinterpret6/1
  Slicer/9(Out9) -> Reinterpret7/1
  Slicer/8(Out8) -> Reinterpret8/1
  Slicer/7(Out7) -> Reinterpret9/1
  Slicer/6(Out6) -> Reinterpret10/1
  Slicer/5(Out5) -> Reinterpret11/1
  Slicer/4(Out4) -> Reinterpret12/1
  Slicer/3(Out3) -> Reinterpret13/1
  Slicer/2(Out2) -> Reinterpret14/1
  Slicer/1(Out1) -> Reinterpret15/1
  Reinterpret/1 -> Gateway Out3/1
  Gateway Out3/1 -> Out16/1
  Reinterpret1/1 -> Gateway Out7/1
  Gateway Out7/1 -> Out15/1
  Reinterpret2/1 -> Gateway Out8/1
  Gateway Out8/1 -> Out14/1
  Reinterpret3/1 -> Gateway Out9/1
  Gateway Out9/1 -> Out13/1
  Reinterpret4/1 -> Gateway Out10/1
  Gateway Out10/1 -> Out12/1
  Reinterpret5/1 -> Gateway Out11/1
  Gateway Out11/1 -> Out11/1
  Reinterpret6/1 -> Gateway Out12/1
  Gateway Out12/1 -> Out10/1
  Reinterpret7/1 -> Gateway Out13/1
  Gateway Out13/1 -> Out9/1
  Reinterpret8/1 -> Gateway Out14/1
  Gateway Out14/1 -> Out8/1
  Reinterpret9/1 -> Gateway Out15/1
  Gateway Out15/1 -> Out7/1
  Reinterpret10/1 -> Gateway Out16/1
  Gateway Out16/1 -> Out6/1
  Reinterpret11/1 -> Gateway Out17/1
  Gateway Out17/1 -> Out5/1
  Reinterpret12/1 -> Gateway Out18/1
  Gateway Out18/1 -> Out4/1
  Reinterpret13/1 -> Gateway Out19/1
  Gateway Out19/1 -> Out3/1
  Reinterpret14/1 -> Gateway Out20/1
  Gateway Out20/1 -> Out2/1
  Reinterpret15/1 -> Gateway Out21/1
  Gateway Out21/1 -> Out1/1

== system dropletdet/BlockAlignment/blk_offset ==
  en : Inport
  Constant : xbsIndex_r4/Constant  const=21-1  gui_display_data_type=Fixed-point  arith_type=Unsigned  n_bits=5  bin_pt=0  preci_type=Single  exp_width=8  frac_width=24  explicit_period=off  period=1  equ=P=C  opselect=C  inp2=PCIN>>17  opr=+  inp1=P  carry=CIN  dbl_ovrd=off  block_type=constant
  Expression : xbsIndex_r4/Expression  expression=a & b  align_bp=on  en=off  latency=0  precision=Full  arith_type=Unsigned  n_bits=16  bin_pt=0  dbl_ovrd=off  block_type=expr
  Relational : xbsIndex_r4/Relational  mode=a=b  en=off  latency=0  dbl_ovrd=off  block_type=relational
  counter_blk_offset1 : xbsIndex_r4/Counter  cnt_type=Free Running  cnt_to=21  operation=Up  start_count=0  cnt_by_val=1  arith_type=Unsigned  n_bits=5  bin_pt=0  load_pin=off  rst=on  en=on  explicit_period=on  period=1  dbl_ovrd=off  use_behavioral_HDL=off  implementation=Fabric  block_type=counter
  eol : Outport
  wires:
  counter_blk_offset1/1 -> Relational/1
  Relational/1 -> Expression/1, counter_blk_offset1/1
  Constant/1 -> Relational/2
  en/1 -> Expression/2, counter_blk_offset1/2
  Expression/1 -> eol/1

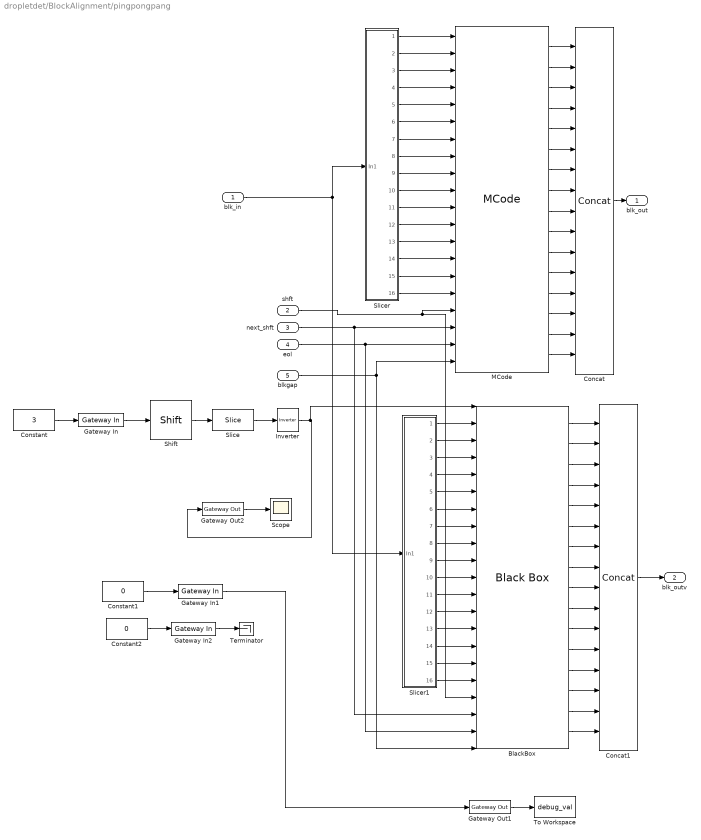
== system dropletdet/BlockAlignment/pingpongpang ==
  blk_in : Inport
  shft : Inport  Port=2
  next_shft : Inport  Port=3
  eol : Inport  Port=4
  blkgap : Inport  Port=5
  BlackBox : xbsIndex_r4/Black Box  init_code=subBlkSelPingPong_config  sim_method=ISE Simulator  verbose=off  block_type=blackbox2
  Concat : xbsIndex_r4/Concat  num_inputs=16  dbl_ovrd=off  block_type=concat
  Concat1 : xbsIndex_r4/Concat  num_inputs=16  dbl_ovrd=off  block_type=concat
  Constant : Constant  Value=3
  Constant1 : Constant  Value=0
  Constant2 : Constant  Value=0
  Gateway In : xbsIndex_r4/Gateway In  gui_display_data_type=Fixed-point  arith_type=Unsigned  n_bits=2  bin_pt=0  preci_type=Single  exp_width=8  frac_width=24  quantization="Round  (unbiased: +/- Inf)"  overflow=Saturate  period=1  dbl_ovrd=off  timing_constraint=None  locs_specified=off  LOCs={}  UseAsADC=off  ADCChannel='1'  inherit_from_input=off  hdl_port=on  block_type=gatewayin
  Gateway In1 : xbsIndex_r4/Gateway In  gui_display_data_type=Fixed-point  arith_type="Signed  (2's comp)"  n_bits=4  bin_pt=0  preci_type=Single  exp_width=8  frac_width=24  quantization="Round  (unbiased: +/- Inf)"  overflow=Saturate  period=1  dbl_ovrd=off  timing_constraint=None  locs_specified=off  LOCs={}  UseAsADC=off  ADCChannel='1'  inherit_from_input=off  hdl_port=on  block_type=gatewayin
  Gateway In2 : xbsIndex_r4/Gateway In  gui_display_data_type=Fixed-point  arith_type="Signed  (2's comp)"  n_bits=1  bin_pt=0  preci_type=Single  exp_width=8  frac_width=24  quantization="Round  (unbiased: +/- Inf)"  overflow=Saturate  period=1  dbl_ovrd=off  timing_constraint=None  locs_specified=off  LOCs={}  UseAsADC=off  ADCChannel='1'  inherit_from_input=off  hdl_port=on  block_type=gatewayin
  Gateway Out1 : xbsIndex_r4/Gateway Out  inherit_from_input=on  hdl_port=off  timing_constraint=None  locs_specified=off  LOCs={}  UseAsDAC=off  DACChannel='1'  block_type=gatewayout
  Gateway Out2 : xbsIndex_r4/Gateway Out  inherit_from_input=off  hdl_port=off  timing_constraint=None  locs_specified=off  LOCs={}  UseAsDAC=off  DACChannel='1'  block_type=gatewayout
  Inverter : xbsIndex_r4/Inverter  en=off  latency=0  dbl_ovrd=off  block_type=inv
  MCode : xbsIndex_r4/MCode  mfname=pingpongpang  explicit_period=off  period=1  inputsTable={'boundInpExpr'=>['','','','','','','','','','','','','','','','','','','',''],'inputs'=>['d15','d14','d13','d12','d11','d10','d09','d08','d07','d06','d05','d04','d03','d02','d01','d00','shft','next_shft','eol','blkgap']}  outputsTable={'outputs'=>['q15','q14','q13','q12','q11','q10','q09','q08','q07','q06','q05','q04','q03','q02','q01','q00'],'suppressOut'=>['off','off','off','off','off','off','off','off','off','off','off','off','off','off','off','off']}  dbl_ovrd=off  enable_stdout=off  enable_debug=off  suppress_output=on  defparams={}  hide_port_list={}  block_type=mcode
  Scope : Scope
  Shift : xbsIndex_r4/Shift  shift_dir=Right  shift_bits=1  en=off  latency=3  precision=Full  arith_type=Unsigned  n_bits=2  bin_pt=0  quantization=Truncate  overflow=Wrap  dbl_ovrd=off  block_type=shift
  Slice : xbsIndex_r4/Slice  nbits=1  boolean_output=on  mode=Lower Bit Location + Width  bit1=0  base1=MSB of Input  bit0=0  base0=LSB of Input  dbl_ovrd=off  block_type=slice
  Slicer : Subsystem
  Slicer1 : Subsystem
  Terminator : Terminator
  To Workspace : ToWorkspace  VariableName=debug_val  SampleTime=-1
  blk_out : Outport
  blk_outv : Outport  Port=2
  wires:
  MCode/14 -> Concat/14
  MCode/15 -> Concat/15
  MCode/16 -> Concat/16
  MCode/1 -> Concat/1
  MCode/2 -> Concat/2
  MCode/3 -> Concat/3
  MCode/4 -> Concat/4
  MCode/5 -> Concat/5
  MCode/6 -> Concat/6
  MCode/8 -> Concat/8
  MCode/7 -> Concat/7
  MCode/12 -> Concat/12
  MCode/13 -> Concat/13
  MCode/9 -> Concat/9
  MCode/10 -> Concat/10
  MCode/11 -> Concat/11
  Concat/1 -> blk_out/1
  Slicer/1(Out1) -> MCode/1
  Slicer/2(Out2) -> MCode/2
  Slicer/3(Out3) -> MCode/3
  Slicer/4(Out4) -> MCode/4
  Slicer/5(Out5) -> MCode/5
  Slicer/6(Out6) -> MCode/6
  Slicer/7(Out7) -> MCode/7
  Slicer/8(Out8) -> MCode/8
  Slicer/9(Out9) -> MCode/9
  Slicer/10(Out10) -> MCode/10
  Slicer/11(Out11) -> MCode/11
  Slicer/12(Out12) -> MCode/12
  Slicer/13(Out13) -> MCode/13
  Slicer/14(Out14) -> MCode/14
  Slicer/15(Out15) -> MCode/15
  Slicer/16(Out16) -> MCode/16
  blk_in/1 -> Slicer1/1(In1), Slicer/1(In1)
  shft/1 -> BlackBox/18, MCode/17
  next_shft/1 -> BlackBox/19, MCode/18
  eol/1 -> BlackBox/20, MCode/19
  blkgap/1 -> BlackBox/21, MCode/20
  Constant/1 -> Gateway In/1
  Constant1/1 -> Gateway In1/1
  Gateway Out1/1 -> To Workspace/1
  Constant2/1 -> Gateway In2/1
  Gateway Out2/1 -> Scope/1
  Shift/1 -> Slice/1
  Gateway In/1 -> Shift/1
  Slice/1 -> Inverter/1
  Inverter/1 -> BlackBox/1, Gateway Out2/1
  Gateway In1/1 -> Gateway Out1/1
  Slicer1/1(Out1) -> BlackBox/2
  Slicer1/2(Out2) -> BlackBox/3
  Slicer1/3(Out3) -> BlackBox/4
  Slicer1/4(Out4) -> BlackBox/5
  Slicer1/5(Out5) -> BlackBox/6
  Slicer1/6(Out6) -> BlackBox/7
  Slicer1/7(Out7) -> BlackBox/8
  Slicer1/8(Out8) -> BlackBox/9
  Slicer1/9(Out9) -> BlackBox/10
  Slicer1/10(Out10) -> BlackBox/11
  Slicer1/11(Out11) -> BlackBox/12
  Slicer1/12(Out12) -> BlackBox/13
  Slicer1/13(Out13) -> BlackBox/14
  Slicer1/14(Out14) -> BlackBox/15
  Slicer1/15(Out15) -> BlackBox/16
  Slicer1/16(Out16) -> BlackBox/17
  BlackBox/16 -> Concat1/16
  BlackBox/15 -> Concat1/15
  BlackBox/14 -> Concat1/14
  BlackBox/13 -> Concat1/13
  BlackBox/12 -> Concat1/12
  BlackBox/11 -> Concat1/11
  BlackBox/10 -> Concat1/10
  BlackBox/9 -> Concat1/9
  BlackBox/8 -> Concat1/8
  BlackBox/7 -> Concat1/7
  BlackBox/6 -> Concat1/6
  BlackBox/5 -> Concat1/5
  BlackBox/4 -> Concat1/4
  BlackBox/3 -> Concat1/3
  BlackBox/2 -> Concat1/2
  BlackBox/1 -> Concat1/1
  Concat1/1 -> blk_outv/1
  Gateway In2/1 -> Terminator/1

== system dropletdet/BlockAlignment/SubBlockAlignment/reg_blkgap ==
  j : Inport
  k : Inport  Port=2
  Expression : xbsIndex_r4/Expression  expression=(~q & j) | (q & ~k)  align_bp=off  en=off  latency=0  precision=Full  arith_type=Unsigned  n_bits=16  bin_pt=0  dbl_ovrd=off  block_type=expr
  Register1 : xbsIndex_r4/Register  init=0  rst=off  en=off  dbl_ovrd=off  block_type=register
  q : Outport
  wires:
  Register1/1 -> Expression/3, q/1
  Expression/1 -> Register1/1
  k/1 -> Expression/2
  j/1 -> Expression/1

== system dropletdet/BlockAlignment/SubSampleAlignment/Fraction ==
  In1 : Inport
  Concat : xbsIndex_r4/Concat  num_inputs=2  dbl_ovrd=off  block_type=concat
  Constant5 : xbsIndex_r4/Constant  const=0  gui_display_data_type=Fixed-point  arith_type=Unsigned  n_bits=2  bin_pt=0  preci_type=Single  exp_width=8  frac_width=24  explicit_period=off  period=1  equ=P=C  opselect=C  inp2=PCIN>>17  opr=+  inp1=P  carry=CIN  dbl_ovrd=off  block_type=constant
  Fractional Part : xbsIndex_r4/Slice  nbits=20  boolean_output=off  mode=Lower Bit Location + Width  bit1=0  base1=MSB of Input  bit0=0  base0=LSB of Input  dbl_ovrd=off  block_type=slice
  Reinterpret : xbsIndex_r4/Reinterpret  force_arith_type=on  arith_type="Signed  (2's comp)"  force_bin_pt=on  bin_pt=20  block_type=reinterpret
  Out1 : Outport
  wires:
  In1/1 -> Fractional Part/1
  Constant5/1 -> Concat/1
  Reinterpret/1 -> Out1/1
  Fractional Part/1 -> Concat/2
  Concat/1 -> Reinterpret/1

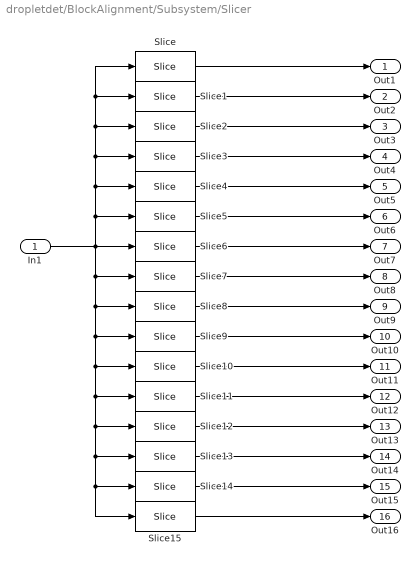
== system dropletdet/BlockAlignment/Subsystem/Slicer ==
  In1 : Inport
  Slice : xbsIndex_r4/Slice  nbits=8  boolean_output=off  mode=Lower Bit Location + Width  bit1=120  base1=MSB of Input  bit0=0  base0=LSB of Input  dbl_ovrd=off  block_type=slice
  Slice1 : xbsIndex_r4/Slice  nbits=8  boolean_output=off  mode=Lower Bit Location + Width  bit1=-8  base1=MSB of Input  bit0=8  base0=LSB of Input  dbl_ovrd=off  block_type=slice
  Slice10 : xbsIndex_r4/Slice  nbits=8  boolean_output=off  mode=Lower Bit Location + Width  bit1=0  base1=MSB of Input  bit0=80  base0=LSB of Input  dbl_ovrd=off  block_type=slice
  Slice11 : xbsIndex_r4/Slice  nbits=8  boolean_output=off  mode=Lower Bit Location + Width  bit1=0  base1=MSB of Input  bit0=88  base0=LSB of Input  dbl_ovrd=off  block_type=slice
  Slice12 : xbsIndex_r4/Slice  nbits=8  boolean_output=off  mode=Lower Bit Location + Width  bit1=0  base1=MSB of Input  bit0=96  base0=LSB of Input  dbl_ovrd=off  block_type=slice
  Slice13 : xbsIndex_r4/Slice  nbits=8  boolean_output=off  mode=Lower Bit Location + Width  bit1=0  base1=MSB of Input  bit0=104  base0=LSB of Input  dbl_ovrd=off  block_type=slice
  Slice14 : xbsIndex_r4/Slice  nbits=8  boolean_output=off  mode=Lower Bit Location + Width  bit1=0  base1=LSB of Input  bit0=112  base0=LSB of Input  dbl_ovrd=off  block_type=slice
  Slice15 : xbsIndex_r4/Slice  nbits=8  boolean_output=off  mode=Lower Bit Location + Width  bit1=0  base1=LSB of Input  bit0=120  base0=LSB of Input  dbl_ovrd=off  block_type=slice
  Slice2 : xbsIndex_r4/Slice  nbits=8  boolean_output=off  mode=Lower Bit Location + Width  bit1=-16  base1=MSB of Input  bit0=16  base0=LSB of Input  dbl_ovrd=off  block_type=slice
  Slice3 : xbsIndex_r4/Slice  nbits=8  boolean_output=off  mode=Lower Bit Location + Width  bit1=-32  base1=MSB of Input  bit0=24  base0=LSB of Input  dbl_ovrd=off  block_type=slice
  Slice4 : xbsIndex_r4/Slice  nbits=8  boolean_output=off  mode=Lower Bit Location + Width  bit1=-40  base1=MSB of Input  bit0=32  base0=LSB of Input  dbl_ovrd=off  block_type=slice
  Slice5 : xbsIndex_r4/Slice  nbits=8  boolean_output=off  mode=Lower Bit Location + Width  bit1=0  base1=MSB of Input  bit0=40  base0=LSB of Input  dbl_ovrd=off  block_type=slice
  Slice6 : xbsIndex_r4/Slice  nbits=8  boolean_output=off  mode=Lower Bit Location + Width  bit1=0  base1=MSB of Input  bit0=48  base0=LSB of Input  dbl_ovrd=off  block_type=slice
  Slice7 : xbsIndex_r4/Slice  nbits=8  boolean_output=off  mode=Lower Bit Location + Width  bit1=0  base1=MSB of Input  bit0=56  base0=LSB of Input  dbl_ovrd=off  block_type=slice
  Slice8 : xbsIndex_r4/Slice  nbits=8  boolean_output=off  mode=Lower Bit Location + Width  bit1=0  base1=MSB of Input  bit0=64  base0=LSB of Input  dbl_ovrd=off  block_type=slice
  Slice9 : xbsIndex_r4/Slice  nbits=8  boolean_output=off  mode=Lower Bit Location + Width  bit1=0  base1=MSB of Input  bit0=72  base0=LSB of Input  dbl_ovrd=off  block_type=slice
  Out1 : Outport
  Out2 : Outport  Port=2
  Out3 : Outport  Port=3
  Out4 : Outport  Port=4
  Out5 : Outport  Port=5
  Out6 : Outport  Port=6
  Out7 : Outport  Port=7
  Out8 : Outport  Port=8
  Out9 : Outport  Port=9
  Out10 : Outport  Port=10
  Out11 : Outport  Port=11
  Out12 : Outport  Port=12
  Out13 : Outport  Port=13
  Out14 : Outport  Port=14
  Out15 : Outport  Port=15
  Out16 : Outport  Port=16
  wires:
  In1/1 -> Slice7/1, Slice8/1, Slice9/1, Slice10/1, Slice11/1, Slice12/1, Slice13/1, Slice14/1, Slice15/1, Slice6/1, Slice5/1, Slice4/1, Slice3/1, Slice2/1, Slice1/1, Slice/1
  Slice1/1 -> Out2/1
  Slice2/1 -> Out3/1
  Slice/1 -> Out1/1
  Slice3/1 -> Out4/1
  Slice4/1 -> Out5/1
  Slice5/1 -> Out6/1
  Slice6/1 -> Out7/1
  Slice7/1 -> Out8/1
  Slice8/1 -> Out9/1
  Slice9/1 -> Out10/1
  Slice10/1 -> Out11/1
  Slice11/1 -> Out12/1
  Slice12/1 -> Out13/1
  Slice13/1 -> Out14/1
  Slice14/1 -> Out15/1
  Slice15/1 -> Out16/1

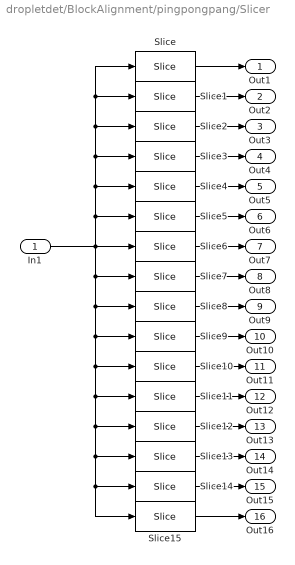
== system dropletdet/BlockAlignment/pingpongpang/Slicer ==
  In1 : Inport
  Slice : xbsIndex_r4/Slice  nbits=8  boolean_output=off  mode=Lower Bit Location + Width  bit1=120  base1=MSB of Input  bit0=120  base0=LSB of Input  dbl_ovrd=off  block_type=slice
  Slice1 : xbsIndex_r4/Slice  nbits=8  boolean_output=off  mode=Lower Bit Location + Width  bit1=-8  base1=MSB of Input  bit0=112  base0=LSB of Input  dbl_ovrd=off  block_type=slice
  Slice10 : xbsIndex_r4/Slice  nbits=8  boolean_output=off  mode=Lower Bit Location + Width  bit1=0  base1=MSB of Input  bit0=40  base0=LSB of Input  dbl_ovrd=off  block_type=slice
  Slice11 : xbsIndex_r4/Slice  nbits=8  boolean_output=off  mode=Lower Bit Location + Width  bit1=0  base1=MSB of Input  bit0=32  base0=LSB of Input  dbl_ovrd=off  block_type=slice
  Slice12 : xbsIndex_r4/Slice  nbits=8  boolean_output=off  mode=Lower Bit Location + Width  bit1=0  base1=MSB of Input  bit0=24  base0=LSB of Input  dbl_ovrd=off  block_type=slice
  Slice13 : xbsIndex_r4/Slice  nbits=8  boolean_output=off  mode=Lower Bit Location + Width  bit1=0  base1=MSB of Input  bit0=16  base0=LSB of Input  dbl_ovrd=off  block_type=slice
  Slice14 : xbsIndex_r4/Slice  nbits=8  boolean_output=off  mode=Lower Bit Location + Width  bit1=0  base1=LSB of Input  bit0=8  base0=LSB of Input  dbl_ovrd=off  block_type=slice
  Slice15 : xbsIndex_r4/Slice  nbits=8  boolean_output=off  mode=Lower Bit Location + Width  bit1=0  base1=LSB of Input  bit0=0  base0=LSB of Input  dbl_ovrd=off  block_type=slice
  Slice2 : xbsIndex_r4/Slice  nbits=8  boolean_output=off  mode=Lower Bit Location + Width  bit1=-16  base1=MSB of Input  bit0=104  base0=LSB of Input  dbl_ovrd=off  block_type=slice
  Slice3 : xbsIndex_r4/Slice  nbits=8  boolean_output=off  mode=Lower Bit Location + Width  bit1=-32  base1=MSB of Input  bit0=96  base0=LSB of Input  dbl_ovrd=off  block_type=slice
  Slice4 : xbsIndex_r4/Slice  nbits=8  boolean_output=off  mode=Lower Bit Location + Width  bit1=-40  base1=MSB of Input  bit0=88  base0=LSB of Input  dbl_ovrd=off  block_type=slice
  Slice5 : xbsIndex_r4/Slice  nbits=8  boolean_output=off  mode=Lower Bit Location + Width  bit1=0  base1=MSB of Input  bit0=80  base0=LSB of Input  dbl_ovrd=off  block_type=slice
  Slice6 : xbsIndex_r4/Slice  nbits=8  boolean_output=off  mode=Lower Bit Location + Width  bit1=0  base1=MSB of Input  bit0=72  base0=LSB of Input  dbl_ovrd=off  block_type=slice
  Slice7 : xbsIndex_r4/Slice  nbits=8  boolean_output=off  mode=Lower Bit Location + Width  bit1=0  base1=MSB of Input  bit0=64  base0=LSB of Input  dbl_ovrd=off  block_type=slice
  Slice8 : xbsIndex_r4/Slice  nbits=8  boolean_output=off  mode=Lower Bit Location + Width  bit1=0  base1=MSB of Input  bit0=56  base0=LSB of Input  dbl_ovrd=off  block_type=slice
  Slice9 : xbsIndex_r4/Slice  nbits=8  boolean_output=off  mode=Lower Bit Location + Width  bit1=0  base1=MSB of Input  bit0=48  base0=LSB of Input  dbl_ovrd=off  block_type=slice
  Out1 : Outport
  Out2 : Outport  Port=2
  Out3 : Outport  Port=3
  Out4 : Outport  Port=4
  Out5 : Outport  Port=5
  Out6 : Outport  Port=6
  Out7 : Outport  Port=7
  Out8 : Outport  Port=8
  Out9 : Outport  Port=9
  Out10 : Outport  Port=10
  Out11 : Outport  Port=11
  Out12 : Outport  Port=12
  Out13 : Outport  Port=13
  Out14 : Outport  Port=14
  Out15 : Outport  Port=15
  Out16 : Outport  Port=16
  wires:
  In1/1 -> Slice7/1, Slice8/1, Slice9/1, Slice10/1, Slice11/1, Slice12/1, Slice13/1, Slice14/1, Slice15/1, Slice6/1, Slice5/1, Slice4/1, Slice3/1, Slice2/1, Slice1/1, Slice/1
  Slice1/1 -> Out2/1
  Slice2/1 -> Out3/1
  Slice/1 -> Out1/1
  Slice3/1 -> Out4/1
  Slice4/1 -> Out5/1
  Slice5/1 -> Out6/1
  Slice6/1 -> Out7/1
  Slice7/1 -> Out8/1
  Slice8/1 -> Out9/1
  Slice9/1 -> Out10/1
  Slice10/1 -> Out11/1
  Slice11/1 -> Out12/1
  Slice12/1 -> Out13/1
  Slice13/1 -> Out14/1
  Slice14/1 -> Out15/1
  Slice15/1 -> Out16/1
